simulink model "moto_linearization"  (R2026a)
settings: Solver=VariableStepAuto  StopTime=30
values from neighbouring files (symbols this model uses):
  ft = bs.FrontTire    [bikeSimToMotoParameters.m]
  Gf = Nsh.'*(Oh - B)    [bikeSimToMotoParameters.m]
  Ib = sum(I,3)    [bikeSimToMotoParameters.m]
  If = sum(I,3)    [bikeSimToMotoParameters.m]
  Ift = zeros(3)    [bikeSimToMotoParameters.m]
  Irt = zeros(3)    [bikeSimToMotoParameters.m]
  m = front_bodies(k).m    [bikeSimToMotoParameters.m]
  N = eye(3)    [bikeSimToMotoParameters.m]
  Ob = sum([rear_bodies.O].*[rear_bodies.m],2)/p.mb    [bikeSimToMotoParameters.m]
  p = motoParameters    [bikeSimToMotoParameters.m]    (also in moto_init.m = bikeSimToPrydeV2Parameters(bs,130/3.6); moto_trim_test.m = P{idx_vx}; steadyTurningTrimEqns.m = in3(41,:); steadyTurningTrimJac.m = in3(41,:))
  pf = fpacejka(bs.FrontTire.Pacejka)    [moto_trim_test.m]
  pr = fpacejka(bs.RearTire.Pacejka)    [moto_trim_test.m]
  rt = bs.RearTire    [bikeSimToMotoParameters.m]
  s = linspace(-pi,pi,36)'    [moto_init.m]
  sm = bs.SprungMass    [bikeSimToMotoParameters.m]
  X = zeros(ns,ns,12)    [moto_trim_test.m]
undefined symbols (not defined in the file or in its folder): mb, mh, Rr, Vlow, Y, Z
libraries: sm_lib x60, nesl_utility x51
(part 1 of 5)
settings Model: Creator=marti  LastModifiedBy=marti
settings ExplorerConfigSet: InternalSimMechanicsExplorerSettings=|
  | <ExplorerConfiguration>
  | 
  |   <canonicalview>default</canonicalview>
  | 
  |   <TilePanel>
  |     <TileInfo>
  |       <Tiles Columns="2" Count="2" Height="610" Rows="1" Width="1503">
  |         <Row Weight="1"/>
  |         <Column Weight="0.5"/>
  |         <Column Weight="0.5"/>
  |         <Tile Height="1" Width="1" X="0" Y="0"/>
  |         <Tile Height="1" Width="1" X="1" Y="0"/>
  |       </Tiles>
  |     </TileInfo>
  |     <SceneInfo>
  |       <SceneViewer>
  |         <IsThisViewStd>
  |           <IsStandardView>off</IsStandardView>
  |           <StandardViewName>Front</StandardViewName>
  |         </IsThisViewStd>
  |         <BGColor>
  |           <R>1</R>
  |           <G>1</G>
  |           <B>1</B>
  |           <A>1</A>
  |         </BGColor>
  |         <Camera>
  |           <DoPerspective>off</DoPerspective>
  |           <Position>
  |             <X>-106.09629365436582</X>
  |             <Y>-2.3701715344858276</Y>
  |             <Z>0.76412826815489532</Z>
  |           </Position>
  |           <Center>
  |             <X>0</X>
  |             <Y>-2.3701715344858276</Y>
  |             <Z>0.76412826815489532</Z>
  |           </Center>
  |           <Up>
  |             <X>0</X>
  |             <Y>0</Y>
  |             <Z>1</Z>
  |           </Up>
  |           <XLim>1.7496107246707635</XLim>
  |           <YLim>1.7496107246707635</YLim>
  |           <ViewLimDist>0.01</ViewLimDist>
  |         </Camera>
  |       </SceneViewer>
  |       <SceneViewer>
  |         <IsThisViewStd>
  |           <IsStandardView>off</IsStandardView>
  |           <StandardViewName>Front</StandardViewName>
  |         </IsThisViewStd>
  |         <BGColor>
  |           <R>1</R>
  |           <G>1</G>
  |           <B>1</B>
  |           <A>1</A>
  |         </BGColor>
  |         <Camera>
  |           <DoPerspective>on</DoPerspective>
  |           <Position>
  |             <X>4.2199890502584978</X>
  |             <Y>-1.5680273619408838</Y>
  |             <Z>0.80000000000000004</Z>
  |           </Position>
  |           <Center>
  |             <X>3.3678925221670628</X>
  |             <Y>-2.0501700213344343</Y>
  |             <Z>0.59635824885982247</Z>
  |           </Center>
  |           <Up>
  |             <X>-0.17723633273196859</X>
  |             <Y>-0.10028581737793676</Y>
  |             <Z>0.97904547248458385</Z>
  |           </Up>
  |           <XLim>0.46630765815499881</XLim>
  |           <YLim>0.46630765815499881</YLim>
  |           <ViewLimDist>0.01</ViewLimDist>
  |         </Camera>
  |       </SceneViewer>
  |     </SceneInfo>
  |   </TilePanel>
  | 
  |   <MechEditorPanel>
  |     <GfxPanelCameraMap>
  |       <MapElement CameraMLId="Camera1" GfxPanelIndex="1"/>
  |     </GfxPanelCameraMap>
  |     <Cameras>
  |       <Camera>
  |         <Id>Camera1</Id>
  |         <Value>
  |           <Name>Camera1</Name>
  |           <NativeCamera>
  |             <PositionTrackingFeature>Subsystem.rear_tire.tracking_camera.F</PositionTrackingFeature>
  |             <CenterTrackingFeature>Subsystem.rear_tire.tracking_camera.F</CenterTrackingFeature>
  |             <UpVectorTrackingFeature>Subsystem.rear_tire.tracking_camera.F</UpVectorTrackingFeature>
  |             <CenterTrackingOrigin>off</CenterTrackingOrigin>
  |             <CenterTrackingDirection>+X</CenterTrackingDirection>
  |             <UpVectorTrackingDirection>+Z</UpVectorTrackingDirection>
  |           </NativeCamera>
  |         </Value>
  |       </Camera>
  |     </Cameras>
  |     <VideoCreator>
  |       <IncludeTiles>All</IncludeTiles>
  |       <IncludeTime>on</IncludeTime>
  |       <IncludeWorldFrame>off</IncludeWorldFrame>
  |       <PlaybackSpeedRatio>1</PlaybackSpeedRatio>
  |       <FrameRate>30</FrameRate>
  |       <FrameSize>auto</FrameSize>
  |       <VideoFormat>UncompressedAVI</VideoFormat>
  |     </VideoCreator>
  |   </MechEditorPanel>
  | 
  |   <PlaybackSettings>
  |     <PlaybackSpeedFactor>4</PlaybackSpeedFactor>
  |   </PlaybackSettings>
  | 
  | </ExplorerConfiguration>

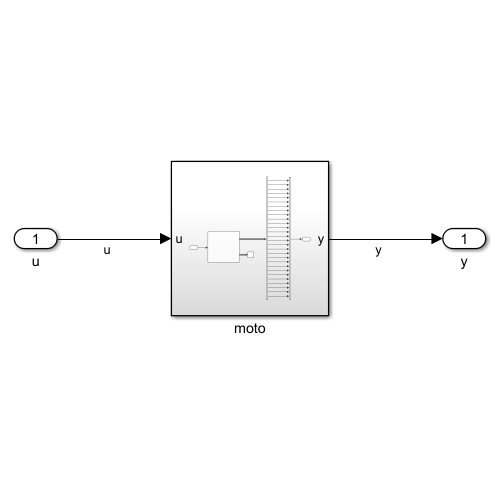
[thumbnail: Simulink's stored preview of the top-level diagram]
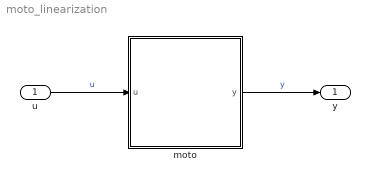
== system moto_linearization ==
  u : Inport
  moto : Subsystem
  y : Outport
  wires:
  u/1 -> moto/1(u)  "u"
  moto/1(y) -> y/1  "y"

== system moto_linearization/moto ==
  u : Inport
  Bus Selector : BusSelector  OutputSignals=RearTire.Position.Yaw,RearTire.Position.X,RearTire.Position.Y,RearTire.Position.Camber,RearTire.Position.Pitch,FrontChassis.Position.Steer,FrontTire.Position.Pitch,RearChassis.Position.Pitch,FrontTire.Position.Yaw,FrontTire.Position.X,FrontTire.Position.Y,FrontTire.Position.Camber,RearTire.Slip.Ratio,FrontTire.Slip.Ratio,RearTire.Slip.Angle,FrontTire.Slip.Angle,RearTire.Velocity.Yaw,RearTire.Velocity.X,RearTire.Velocity.Y,RearTire.Velocity.Camber,RearTire.Velocity.Pitch,FrontChassis.Velocity.Steer,FrontTire.Velocity.Pitch,RearChassis.Velocity.Pitch,FrontTire.Velocity.Yaw,FrontTire.Velocity.X,FrontTire.Velocity.Y,FrontTire.Velocity.Camber
  Mux : Mux  Inputs=28
  Subsystem : Subsystem
  Terminator : Terminator
  y : Outport
  wires:
  u/1 -> Subsystem/1(u)
  Subsystem/2(Control) -> Terminator/1
  Subsystem/1(Info) -> Bus Selector/1
  Bus Selector/1 -> Mux/1  "<Yaw>"
  Bus Selector/2 -> Mux/2  "<X>"
  Bus Selector/3 -> Mux/3  "<Y>"
  Bus Selector/4 -> Mux/4  "<Camber>"
  Bus Selector/5 -> Mux/5  "<Pitch>"
  Bus Selector/6 -> Mux/6  "<Steer>"
  Bus Selector/7 -> Mux/7  "<Pitch>"
  Bus Selector/8 -> Mux/8  "<Pitch>"
  Bus Selector/9 -> Mux/9  "<Yaw>"
  Bus Selector/10 -> Mux/10  "<X>"
  Bus Selector/11 -> Mux/11  "<Y>"
  Bus Selector/12 -> Mux/12  "<Camber>"
  Bus Selector/13 -> Mux/13  "<Ratio>"
  Bus Selector/14 -> Mux/14  "<Ratio>"
  Bus Selector/15 -> Mux/15  "<Angle>"
  Bus Selector/16 -> Mux/16  "<Angle>"
  Bus Selector/17 -> Mux/17  "<Yaw>"
  Bus Selector/18 -> Mux/18  "<X>"
  Bus Selector/19 -> Mux/19  "<Y>"
  Bus Selector/20 -> Mux/20  "<Camber>"
  Bus Selector/21 -> Mux/21  "<Pitch>"
  Bus Selector/22 -> Mux/22  "<Steer>"
  Bus Selector/23 -> Mux/23  "<Pitch>"
  Bus Selector/24 -> Mux/24  "<Pitch>"
  Bus Selector/25 -> Mux/25  "<Yaw>"
  Bus Selector/26 -> Mux/26  "<X>"
  Bus Selector/27 -> Mux/27  "<Y>"
  Bus Selector/28 -> Mux/28  "<Camber>"
  Mux/1 -> y/1

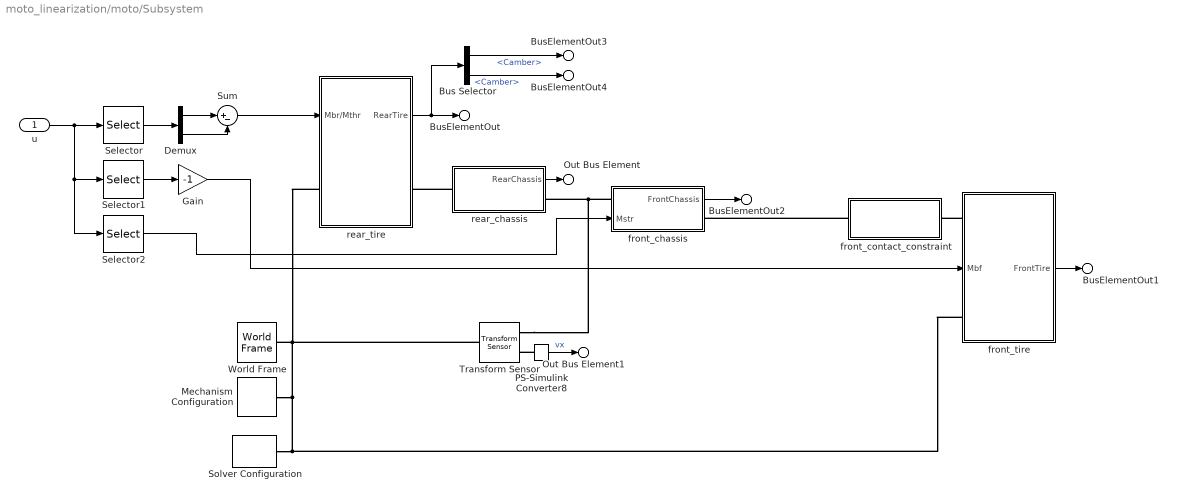
== system moto_linearization/moto/Subsystem ==
  u : Inport
  Bus Selector : BusSelector  OutputSignals=Position.Camber,Velocity.Camber
  Demux : Demux  Outputs=2
  Gain : Gain  Gain=-1
  Mechanism Configuration : sm_lib/Utilities/Mechanism Configuration  UniformGravity=Constant  GravityVector=[0 0 -p.g]  GravityVectorUnits=m/s^2  LinearizationDelta=0.001  JointModeTransitionNonlinearIterations=2
  PS-Simulink Converter8 : nesl_utility/PS-Simulink Converter  PhysicalDomain=network_engine_domain  SubClassName=ps_output  LeftPortType=input  RightPortType=output  PseudoPeriodic=off  Frequencies=[]  VectorFormat=inherit  Unit=inherit  AffineConversion=off
  Selector : Selector  InputPortWidth=4  IndexOptions=Index vector (dialog)  Indices=1:2  OutputSizes=1
  Selector1 : Selector  InputPortWidth=4  IndexOptions=Index vector (dialog)  Indices=3  OutputSizes=1
  Selector2 : Selector  InputPortWidth=4  IndexOptions=Index vector (dialog)  Indices=4  OutputSizes=1
  Solver Configuration : nesl_utility/Solver Configuration  PhysicalDomain=network_engine_domain  SubClassName=solver  LeftPortType=input  RightPortType=generic  Tones=[]  Harmonics=[]  SimulateNoise=off  Profile=off  UseLocalSampling=off  EnableSwitchedLinearOptims=on  FrequencyDomain=off  UseCCode=off  RelTol=0.001  AbsTol=0.001  MinStep=1e-09  ToWorkspace=off  RevertToSquareIcSolve=off  NumHomotopyIterations=100  PhasorMode=off  PhasorModeNumHarmonics=1  ConsistencySolver=NEWTON_XTOL_AFTER_FTOL  CanonicalOrdering=CANONICAL  OptimizeIntermediates=OPTIMIZED  IndexReductionMethod=DerivativeReplacement  DoDC=off  ResidualTolerance=1e-09  ConsistencyTolSource=GLOBAL  ConsistencyAbsTol=0.001  ConsistencyRelTol=0.001  ConsistencyTolFactor=0.001  UseLocalSolver=off  LocalSolverChoice=NE_BACKWARD_EULER_ADVANCER  ResolveIndetEquations=on  FunctionEvalNumThread=1  LocalSolverSampleTime=0.001  DoFixedCost=off  MaxNonlinIter=3  MaxModeIter=2  ComputeImpulses=off  ImpulseIterations=2  LinearAlgebra=auto  LinearAlgebraNumThread=0  EquationFormulation=NE_TIME_EF  DelaysMemoryBudget=1024  AutomaticFiltering=on  FilteringTimeConstant=0.001  PartitionStorageMethod=AS_NEEDED  PartitionMemoryBudget=1024  PartitionMethod=ROBUST  MultibodyUseLocalSolver=off  MultibodyLocalSolverChoice=ODE1  MultibodyLocalSolverSampleTime=0.001
  Sum : Sum  Inputs=|+-
  Transform Sensor : sm_lib/Frames and Transforms/Transform Sensor  MeasurementFrame=NonRotatingFollower  RotationSequence=ZXY  SenseAngle=off  SenseAxis=off  SenseQ=off  SenseR=off  SenseRotationSequence=off  SenseOmegaX=off  SenseOmegaY=off  SenseOmegaZ=off  SenseOmega=off  SenseQDot=off  SenseRDot=off  SenseRotationSequenceDot=off  SenseAlphaX=off  SenseAlphaY=off  SenseAlphaZ=off  SenseAlpha=off  SenseQDDot=off  SenseRDDot=off  SenseX=off  SenseY=off  SenseZ=off  SenseXYZ=off  SenseRad=off  SenseAzim=off  SenseDist=off  SenseInc=off  SenseXDot=on  SenseYDot=off  SenseZDot=off  SenseXYZDot=off  SenseRadDot=off  SenseAzimDot=off  SenseDistDot=off  SenseIncDot=off  SenseXDDot=off  SenseYDDot=off  SenseZDDot=off  SenseXYZDDot=off  SenseRadDDot=off  SenseAzimDDot=off  SenseDistDDot=off  SenseIncDDot=off
  World Frame : sm_lib/Frames and Transforms/World Frame
  front_chassis : Subsystem
      settings: PortSchema="{\"entries\":[{\"content\":{\"sides\":[{\"content\":{\"connectorIds\":[\"LConn1\",\"In1\"]},\"type\":\"ConnectorPlacement.EquallySpacedRectSide\",\"uuid\":\"28cd6f4b-604a-4bcb-85e2-114c9cc0d3d3\"},{\"content\":{\"connectorIds\":[\"Out1\",\"RConn1\"],\"side\":\"RIGHT\"},\"type\":\"ConnectorPlacement.EquallySpacedRectSide\",\"uuid\":\"84947a28-75e1-48cb-906c-17d8aa3b8f8d\"},{\"content\":{\"side\":\"TOP\"},\"type\":\"ConnectorPlacement.EquallySpacedRectSide\",\"uuid\":\"c08a0e8d-a466-4273-a35e-c448cbe89ae5\"}]},\"type\":\"ConnectorPlacement.EquallySpacedConnector\",\"uuid\":\"52103cf8-afef-4fdc-bf57-92bfaf3948ff\"}],\"packageUris\":[\"http://schema.mathworks.com/mf0/Connector/R2020b\"],\"version\":\"1.0\"}"
  front_contact_constraint : Subsystem
  front_tire : Subsystem
      settings: PortSchema="{\"entries\":[{\"content\":{\"sides\":[{\"content\":{\"connectorIds\":[\"LConn1\",\"In1\",\"LConn2\"]},\"type\":\"ConnectorPlacement.EquallySpacedRectSide\",\"uuid\":\"28cd6f4b-604a-4bcb-85e2-114c9cc0d3d3\"},{\"content\":{\"connectorIds\":[\"Out1\"],\"side\":\"RIGHT\"},\"type\":\"ConnectorPlacement.EquallySpacedRectSide\",\"uuid\":\"84947a28-75e1-48cb-906c-17d8aa3b8f8d\"},{\"content\":{\"side\":\"TOP\"},\"type\":\"ConnectorPlacement.EquallySpacedRectSide\",\"uuid\":\"c08a0e8d-a466-4273-a35e-c448cbe89ae5\"}]},\"type\":\"ConnectorPlacement.EquallySpacedConnector\",\"uuid\":\"52103cf8-afef-4fdc-bf57-92bfaf3948ff\"}],\"packageUris\":[\"http://schema.mathworks.com/mf0/Connector/R2020b\"],\"version\":\"1.0\"}"
  rear_chassis : Subsystem
  rear_tire : Subsystem
  BusElementOut : Outport  PortName=Info  Element=RearTire
  Out Bus Element : Outport  PortName=Info  Element=RearChassis
  BusElementOut2 : Outport  PortName=Info  Element=FrontChassis
  BusElementOut1 : Outport  PortName=Info  Element=FrontTire
  Out Bus Element1 : Outport  Port=2  PortName=Control  Element=Vx
  BusElementOut3 : Outport  Port=2  PortName=Control  Element=Camber
  BusElementOut4 : Outport  Port=2  PortName=Control  Element=CamberRate
  wires:
  rear_chassis/1(RearChassis) -> Out Bus Element/1
  rear_tire/1(RearTire) -> Bus Selector/1, BusElementOut/1
  front_chassis/1(FrontChassis) -> BusElementOut2/1
  front_tire/1(FrontTire) -> BusElementOut1/1
  PS-Simulink Converter8/1 -> Out Bus Element1/1  "vx"
  Bus Selector/1 -> BusElementOut3/1  "<Camber>"
  Bus Selector/2 -> BusElementOut4/1  "<Camber>"
  u/1 -> Selector2/1, Selector1/1, Selector/1
  Selector/1 -> Demux/1
  Demux/1 -> Sum/1
  Demux/2 -> Sum/2
  Sum/1 -> rear_tire/1(Mbr/Mthr)
  Selector1/1 -> Gain/1
  Gain/1 -> front_tire/1(Mbf)
  Selector2/1 -> front_chassis/1(Mstr)
  connections:
  front_chassis/LConn1 -- Transform Sensor/RConn1 -- rear_chassis/RConn1
  Solver Configuration/RConn1 -- rear_tire/LConn1 -- Transform Sensor/LConn1 -- World Frame/RConn1 -- Mechanism Configuration/RConn1 -- front_tire/LConn2
  front_contact_constraint/RConn1 -- front_chassis/RConn1
  rear_chassis/LConn1 -- rear_tire/RConn1
  front_tire/LConn1 -- front_contact_constraint/LConn1
  PS-Simulink Converter8/LConn1 -- Transform Sensor/RConn2

== system moto_linearization/moto/Subsystem/front_chassis ==
  Mstr : Inport
  " f" : sm_lib/Frames and Transforms/Rigid Transform  RotationMethod=None  FollAlignAxisA=+X  BaseAlignAxisA=+Y  FollAlignAxisB=+Y  BaseAlignAxisB=+Z  RotationStandardAxis=+Z  RotationAngle=0  RotationAngleUnits=deg  RotationArbitraryAxis=[0 0 1]  RotationSequenceAxes=FollowerAxes  RotationSequence=XYX  RotationSequenceAngles=[0 0 0]  RotationSequenceAnglesUnits=deg  RotationMatrix=[1 0 0;0 1 0;0 0 1]  Quaternion=[1 0 0 0]  TranslationMethod=StandardAxis  TranslationCartesianOffset=[0 0 0]  TranslationCartesianOffsetUnits=m  TranslationStandardAxis=+Z  TranslationStandardOffset=Gf(3)  TranslationStandardOffsetUnits=m  TranslationROffset=0  TranslationROffsetUnits=m  TranslationThetaOffset=0  TranslationThetaOffsetUnits=deg  TranslationZOffset=0  TranslationZOffsetUnits=m
  PS-Simulink Converter1 : nesl_utility/PS-Simulink Converter  PhysicalDomain=network_engine_domain  SubClassName=ps_output  LeftPortType=input  RightPortType=output  PseudoPeriodic=off  Frequencies=[]  VectorFormat=inherit  Unit=inherit  AffineConversion=off
  PS-Simulink Converter2 : nesl_utility/PS-Simulink Converter  PhysicalDomain=network_engine_domain  SubClassName=ps_output  LeftPortType=input  RightPortType=output  PseudoPeriodic=off  Frequencies=[]  VectorFormat=inherit  Unit=inherit  AffineConversion=off
  PS-Simulink Converter4 : nesl_utility/PS-Simulink Converter  PhysicalDomain=network_engine_domain  SubClassName=ps_output  LeftPortType=input  RightPortType=output  PseudoPeriodic=off  Frequencies=[]  VectorFormat=inherit  Unit=inherit  AffineConversion=off
  Simulink-PS Converter2 : nesl_utility/Simulink-PS Converter  PhysicalDomain=network_engine_domain  SubClassName=ps_input  LeftPortType=input  RightPortType=output  PseudoPeriodic=off  Frequencies=[]  NoiseDistribution=none  NoiseParameters=[]  Unit=N*m  AffineConversion=off  FilteringAndDerivatives=provide  SimscapeFilterOrder=1  InputFilterTimeConstant=0.001  UdotUserProvided=0
  caster : sm_lib/Frames and Transforms/Rigid Transform  RotationMethod=StandardAxis  FollAlignAxisA=+X  BaseAlignAxisA=+Y  FollAlignAxisB=+Y  BaseAlignAxisB=+Z  RotationStandardAxis=-Y  RotationAngle=caster  RotationAngleUnits=rad  RotationArbitraryAxis=[0 0 1]  RotationSequenceAxes=FollowerAxes  RotationSequence=XYX  RotationSequenceAngles=[0 0 0]  RotationSequenceAnglesUnits=deg  RotationMatrix=[1 0 0;0 1 0;0 0 1]  Quaternion=[1 0 0 0]  TranslationMethod=None  TranslationCartesianOffset=[0 0 0]  TranslationCartesianOffsetUnits=m  TranslationStandardAxis=+Z  TranslationStandardOffset=0  TranslationStandardOffsetUnits=m  TranslationROffset=0  TranslationROffsetUnits=m  TranslationThetaOffset=0  TranslationThetaOffsetUnits=deg  TranslationZOffset=0  TranslationZOffsetUnits=m
  chord : sm_lib/Frames and Transforms/Rigid Transform  RotationMethod=None  FollAlignAxisA=+X  BaseAlignAxisA=+Y  FollAlignAxisB=+Y  BaseAlignAxisB=+Z  RotationStandardAxis=+Z  RotationAngle=0  RotationAngleUnits=deg  RotationArbitraryAxis=[0 0 1]  RotationSequenceAxes=FollowerAxes  RotationSequence=XYX  RotationSequenceAngles=[0 0 0]  RotationSequenceAnglesUnits=deg  RotationMatrix=[1 0 0;0 1 0;0 0 1]  Quaternion=[1 0 0 0]  TranslationMethod=StandardAxis  TranslationCartesianOffset=[0 0 0]  TranslationCartesianOffsetUnits=m  TranslationStandardAxis=+X  TranslationStandardOffset=a  TranslationStandardOffsetUnits=m  TranslationROffset=0  TranslationROffsetUnits=m  TranslationThetaOffset=0  TranslationThetaOffsetUnits=deg  TranslationZOffset=0  TranslationZOffsetUnits=m
  e : sm_lib/Frames and Transforms/Rigid Transform  RotationMethod=None  FollAlignAxisA=+X  BaseAlignAxisA=+Y  FollAlignAxisB=+Y  BaseAlignAxisB=+Z  RotationStandardAxis=+Z  RotationAngle=0  RotationAngleUnits=deg  RotationArbitraryAxis=[0 0 1]  RotationSequenceAxes=FollowerAxes  RotationSequence=XYX  RotationSequenceAngles=[0 0 0]  RotationSequenceAnglesUnits=deg  RotationMatrix=[1 0 0;0 1 0;0 0 1]  Quaternion=[1 0 0 0]  TranslationMethod=StandardAxis  TranslationCartesianOffset=[0 0 0]  TranslationCartesianOffsetUnits=m  TranslationStandardAxis=+X  TranslationStandardOffset=Gf(1)  TranslationStandardOffsetUnits=m  TranslationROffset=0  TranslationROffsetUnits=m  TranslationThetaOffset=0  TranslationThetaOffsetUnits=deg  TranslationZOffset=0  TranslationZOffsetUnits=m
  front_chassis : sm_lib/Body Elements/File Solid  ExtGeomFileName=front_chassis.stl  UnitType=Custom  ExtGeomFileUnits=mm  StepReaderType=HEX  ExportConvexHullGeometry=off  InertiaType=Custom  BasedOnType=DensityFromFile  Density=1000  DensityUnits=kg/m^3  Mass=mh  MassUnits=kg  CenterOfMass=[0 0 0]  CenterOfMassUnits=m  MomentsOfInertia=diag(If)  MomentsOfInertiaUnits=kg*m^2  ProductsOfInertia=[0 If(1,3) 0]  ProductsOfInertiaUnits=kg*m^2  GraphicType=FromGeometry  MarkerShape=Sphere  MarkerSize=10  GraphicVisPropType=SimpleVisualProperties  GraphicDiffuseColor=[1 0 0]  GraphicOpacity=1  GraphicSpecularColor=[0.5 0.5 0.5 1.0]  GraphicAmbientColor=[0.15 0.15 0.15 1.0]  GraphicEmissiveColor=[0.0 0.0 0.0 1.0]  GraphicShininess=75  DoExposeReferenceFrame=on  SerializedFrames=<Frames/>
  lz : sm_lib/Frames and Transforms/Rigid Transform  RotationMethod=None  FollAlignAxisA=+X  BaseAlignAxisA=+Y  FollAlignAxisB=+Y  BaseAlignAxisB=+Z  RotationStandardAxis=+Z  RotationAngle=0  RotationAngleUnits=deg  RotationArbitraryAxis=[0 0 1]  RotationSequenceAxes=FollowerAxes  RotationSequence=XYX  RotationSequenceAngles=[0 0 0]  RotationSequenceAnglesUnits=deg  RotationMatrix=[1 0 0;0 1 0;0 0 1]  Quaternion=[1 0 0 0]  TranslationMethod=StandardAxis  TranslationCartesianOffset=[0 0 0]  TranslationCartesianOffsetUnits=m  TranslationStandardAxis=-Z  TranslationStandardOffset=lz  TranslationStandardOffsetUnits=m  TranslationROffset=0  TranslationROffsetUnits=m  TranslationThetaOffset=0  TranslationThetaOffsetUnits=deg  TranslationZOffset=0  TranslationZOffsetUnits=m
  rake : sm_lib/Frames and Transforms/Rigid Transform  RotationMethod=None  FollAlignAxisA=+X  BaseAlignAxisA=+Y  FollAlignAxisB=+Y  BaseAlignAxisB=+Z  RotationStandardAxis=+Z  RotationAngle=0  RotationAngleUnits=deg  RotationArbitraryAxis=[0 0 1]  RotationSequenceAxes=FollowerAxes  RotationSequence=XYX  RotationSequenceAngles=[0 0 0]  RotationSequenceAnglesUnits=deg  RotationMatrix=[1 0 0;0 1 0;0 0 1]  Quaternion=[1 0 0 0]  TranslationMethod=StandardAxis  TranslationCartesianOffset=[0 0 0]  TranslationCartesianOffsetUnits=m  TranslationStandardAxis=+X  TranslationStandardOffset=sh.Rake  TranslationStandardOffsetUnits=m  TranslationROffset=0  TranslationROffsetUnits=m  TranslationThetaOffset=0  TranslationThetaOffsetUnits=deg  TranslationZOffset=0  TranslationZOffsetUnits=m
  steer_joint : sm_lib/Joints/Revolute Joint  JointMode=Normal  CompositeWrenchDir=FollowerOnBase  CompositeWrenchFrame=BaseFrame  SenseConstraintForce=off  SenseConstraintTorque=off  SenseTotalForce=off  SenseTotalTorque=off  PositionTargetSpecify=off  PositionTargetPriority=High  PositionTargetValue=0  PositionTargetValueUnits=deg  VelocityTargetSpecify=off  VelocityTargetPriority=High  VelocityTargetValue=0  VelocityTargetValueUnits=deg/s  EquilibriumPosition=0  EquilibriumPositionUnits=deg  SpringStiffness=0  SpringStiffnessUnits=N*m/deg  DampingCoefficient=sh.Damping  DampingCoefficientUnits=N*m/(deg/s)  LowerLimitSpecify=off  LowerLimitBound=-90  LowerLimitBoundUnits=deg  LowerLimitStiffness=1e4  LowerLimitStiffnessUnits=N*m/deg  LowerLimitDamping=10  LowerLimitDampingUnits=N*m/(deg/s)  LowerLimitTransitionRegionWidth=0.1  LowerLimitTransitionRegionWidthUnits=deg  UpperLimitSpecify=off  UpperLimitBound=90  UpperLimitBoundUnits=deg  UpperLimitStiffness=1e4  UpperLimitStiffnessUnits=N*m/deg  UpperLimitDamping=10  UpperLimitDampingUnits=N*m/(deg/s)  UpperLimitTransitionRegionWidth=0.1  UpperLimitTransitionRegionWidthUnits=deg  TorqueActuationMode=InputTorque  MotionActuationMode=ComputedMotion  SensePosition=on  SenseVelocity=on  SenseAcceleration=on  SenseTorqueForce=off  SenseLowerLimitTorqueForce=off  SenseUpperLimitTorqueForce=off
  B : PMIOPort  Side=Left
  F : PMIOPort  Port=2  Side=Right
  BusElementOut : Outport  PortName=FrontChassis  Element=Position.Steer
  BusElementOut1 : Outport  PortName=FrontChassis  Element=Velocity.Steer
  BusElementOut2 : Outport  PortName=FrontChassis  Element=Acceleration.Steer
  wires:
  Mstr/1 -> Simulink-PS Converter2/1  "Mstr"
  PS-Simulink Converter4/1 -> BusElementOut/1  "steer"
  PS-Simulink Converter1/1 -> BusElementOut1/1  "dsteer"
  PS-Simulink Converter2/1 -> BusElementOut2/1  "ddsteer"
  connections:
  e/LConn1 -- lz/LConn1 -- rake/RConn1
  " f"/LConn1 -- e/RConn1
  Simulink-PS Converter2/RConn1 -- steer_joint/LConn2
  front_chassis/RConn1 -- " f"/RConn1
  chord/RConn1 -- steer_joint/LConn1
  PS-Simulink Converter4/LConn1 -- steer_joint/RConn2
  chord/LConn1 -- caster/RConn1
  rake/LConn1 -- steer_joint/RConn1
  lz/RConn1 -- F/RConn1
  caster/LConn1 -- B/RConn1
  PS-Simulink Converter1/LConn1 -- steer_joint/RConn3
  steer_joint/RConn4 -- PS-Simulink Converter2/LConn1

== system moto_linearization/moto/Subsystem/front_contact_constraint ==
  Rigid Transform20 : sm_lib/Frames and Transforms/Rigid Transform  RotationMethod=StandardAxis  FollAlignAxisA=+X  BaseAlignAxisA=+Y  FollAlignAxisB=+Y  BaseAlignAxisB=+Z  RotationStandardAxis=-X  RotationAngle=90  RotationAngleUnits=deg  RotationArbitraryAxis=[0 0 1]  RotationSequenceAxes=FollowerAxes  RotationSequence=XYX  RotationSequenceAngles=[0 0 0]  RotationSequenceAnglesUnits=deg  RotationMatrix=[1 0 0;0 1 0;0 0 1]  Quaternion=[1 0 0 0]  TranslationMethod=None  TranslationCartesianOffset=[0 0 0]  TranslationCartesianOffsetUnits=m  TranslationStandardAxis=+Z  TranslationStandardOffset=0  TranslationStandardOffsetUnits=m  TranslationROffset=0  TranslationROffsetUnits=m  TranslationThetaOffset=0  TranslationThetaOffsetUnits=deg  TranslationZOffset=0  TranslationZOffsetUnits=m
  Rigid Transform21 : sm_lib/Frames and Transforms/Rigid Transform  RotationMethod=StandardAxis  FollAlignAxisA=+X  BaseAlignAxisA=+Y  FollAlignAxisB=+Y  BaseAlignAxisB=+Z  RotationStandardAxis=+X  RotationAngle=90  RotationAngleUnits=deg  RotationArbitraryAxis=[0 0 1]  RotationSequenceAxes=FollowerAxes  RotationSequence=XYX  RotationSequenceAngles=[0 0 0]  RotationSequenceAnglesUnits=deg  RotationMatrix=[1 0 0;0 1 0;0 0 1]  Quaternion=[1 0 0 0]  TranslationMethod=None  TranslationCartesianOffset=[0 0 0]  TranslationCartesianOffsetUnits=m  TranslationStandardAxis=+Z  TranslationStandardOffset=0  TranslationStandardOffsetUnits=m  TranslationROffset=0  TranslationROffsetUnits=m  TranslationThetaOffset=0  TranslationThetaOffsetUnits=deg  TranslationZOffset=0  TranslationZOffsetUnits=m
  caster : sm_lib/Frames and Transforms/Rigid Transform  RotationMethod=StandardAxis  FollAlignAxisA=+X  BaseAlignAxisA=+Y  FollAlignAxisB=+Y  BaseAlignAxisB=+Z  RotationStandardAxis=+Y  RotationAngle=caster  RotationAngleUnits=rad  RotationArbitraryAxis=[0 0 1]  RotationSequenceAxes=FollowerAxes  RotationSequence=XYX  RotationSequenceAngles=[0 0 0]  RotationSequenceAnglesUnits=deg  RotationMatrix=[1 0 0;0 1 0;0 0 1]  Quaternion=[1 0 0 0]  TranslationMethod=None  TranslationCartesianOffset=[0 0 0]  TranslationCartesianOffsetUnits=m  TranslationStandardAxis=+Z  TranslationStandardOffset=0  TranslationStandardOffsetUnits=m  TranslationROffset=0  TranslationROffsetUnits=m  TranslationThetaOffset=0  TranslationThetaOffsetUnits=deg  TranslationZOffset=0  TranslationZOffsetUnits=m
  reach_joint : sm_lib/Joints/Revolute Joint  JointMode=Normal  CompositeWrenchDir=FollowerOnBase  CompositeWrenchFrame=BaseFrame  SenseConstraintForce=off  SenseConstraintTorque=off  SenseTotalForce=off  SenseTotalTorque=off  PositionTargetSpecify=off  PositionTargetPriority=High  PositionTargetValue=0  PositionTargetValueUnits=deg  VelocityTargetSpecify=off  VelocityTargetPriority=High  VelocityTargetValue=0  VelocityTargetValueUnits=deg/s  EquilibriumPosition=0  EquilibriumPositionUnits=deg  SpringStiffness=0  SpringStiffnessUnits=N*m/deg  DampingCoefficient=0  DampingCoefficientUnits=N*m/(deg/s)  LowerLimitSpecify=off  LowerLimitBound=-90  LowerLimitBoundUnits=deg  LowerLimitStiffness=1e4  LowerLimitStiffnessUnits=N*m/deg  LowerLimitDamping=10  LowerLimitDampingUnits=N*m/(deg/s)  LowerLimitTransitionRegionWidth=0.1  LowerLimitTransitionRegionWidthUnits=deg  UpperLimitSpecify=off  UpperLimitBound=90  UpperLimitBoundUnits=deg  UpperLimitStiffness=1e4  UpperLimitStiffnessUnits=N*m/deg  UpperLimitDamping=10  UpperLimitDampingUnits=N*m/(deg/s)  UpperLimitTransitionRegionWidth=0.1  UpperLimitTransitionRegionWidthUnits=deg  TorqueActuationMode=NoTorque  MotionActuationMode=ComputedMotion  SensePosition=off  SenseVelocity=off  SenseAcceleration=off  SenseTorqueForce=off  SenseLowerLimitTorqueForce=off  SenseUpperLimitTorqueForce=off
  F : PMIOPort  Side=Right
  B : PMIOPort  Port=2  Side=Left
  connections:
  Rigid Transform21/LConn1 -- reach_joint/RConn1
  Rigid Transform20/RConn1 -- reach_joint/LConn1
  Rigid Transform21/RConn1 -- caster/LConn1
  Rigid Transform20/LConn1 -- B/RConn1
  caster/RConn1 -- F/RConn1
